simulink model "gps_casestudy_1_2"  (R2023a)
settings: Solver=VariableStepAuto  StartTime=0.0  StopTime=10  RelTol=1e-3
settings Model: PacingRate=0.890000  Creator=simon  LastModifiedBy=simon

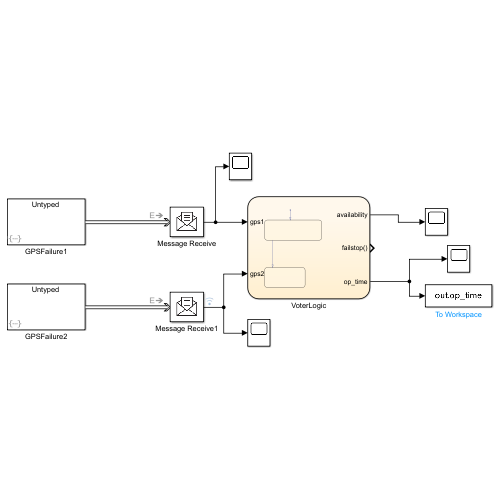
[thumbnail: Simulink's stored preview of the top-level diagram]
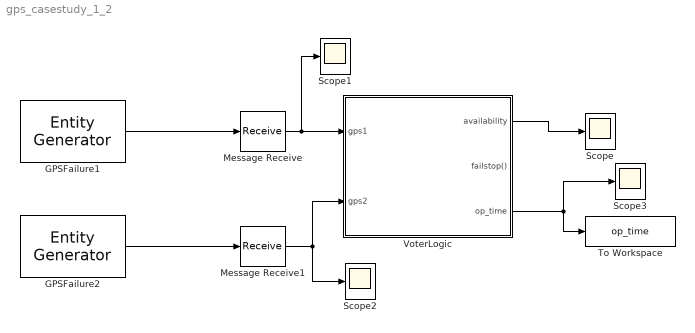
== system gps_casestudy_1_2 ==
  GPSFailure1 : EntityGenerator  OutputPortMessageModes=m  TimeSource=MATLAB action  IntergenerationTimeAction=dt = -14.1*log(1-rand());  GenerateEntityAtSimulationStart=off  GenerateAction=entity=0;  AttributeName=entity  EntityTypeName=GPS1FailureGenerator  DataInitialValue=1
  GPSFailure2 : EntityGenerator  OutputPortMessageModes=m  TimeSource=MATLAB action  IntergenerationTimeAction=dt = -14.1*log(1-rand());  GenerateEntityAtSimulationStart=off  GenerateAction=entity=0;  AttributeName=entity  EntityTypeName=GPS1FailureGenerator  DataInitialValue=1
  Message Receive : Receive  InputPortMessageModes=m  QueueLength=1  InitialValue=[1]
  Message Receive1 : Receive  InputPortMessageModes=m  QueueLength=1  InitialValue=[1]
  Scope{,1..3} (4 alike) : Scope
  To Workspace : ToWorkspace  VariableName=op_time  SaveFormat=Timeseries  SampleTime=-1
  VoterLogic : Stateflow chart  TreatAsAtomicUnit=on
      settings: PortSchema="{\"entries\":[{\"content\":{\"sides\":[{\"content\":{\"connectorIds\":[\"In1\",\"In2\"]},\"type\":\"ConnectorPlacement.EquallySpacedRectSide\",\"uuid\":\"ade0a091-17ce-42a4-aa78-d0bfb30748c5\"},{\"content\":{\"connectorIds\":[\"Out1\",\"Out3\",\"Out2\"],\"side\":\"RIGHT\"},\"type\":\"ConnectorPlacement.EquallySpacedRectSide\",\"uuid\":\"66555fcb-1f83-4e30-8ef8-6a8313a50ee1\"},{\"content\":{\"side\":\"TOP\"},\"type\":\"ConnectorPlacement.EquallySpacedRectSide\",\"uuid\":\"cf416699-892d-4ad5-b2c8-eaa41a09f8ad\"}]},\"type\":\"ConnectorPlacement.EquallySpacedConnector\",\"uuid\":\"2c45de72-65a5-4ed7-b40b-303d32fb903d\"}],\"packageUris\":[\"http://schema.mathworks.com/mf0/Connector/R2020b\"],\"version\":\"1.0\"}"
  wires:
  GPSFailure1/1 -> Message Receive/1
  GPSFailure2/1 -> Message Receive1/1
  VoterLogic/1(availability) -> Scope/1
  Message Receive/1 -> Scope1/1, VoterLogic/1(gps1)
  Message Receive1/1 -> Scope2/1, VoterLogic/2(gps2)
  VoterLogic/2(op_time) -> To Workspace/1, Scope3/1

== stateflow chart gps_casestudy_1_2/VoterLogic ==
  settings: sampleTime=0.01  executeAtInitialization=1
  state Operation
    exit:
    op_time=temporalCount(sec)
  state Failstop
  (default) -> Operation : {availability=1}
  Operation -> Failstop : [(gps1==0) && (gps2==0)]{availability=0;send(failstop);}
  data: availability output; gps1 input; gps2 input; op_time output
  events: failstop output FUNCTION_CALL_EVENT
